simulink subsystem "SubFaultGate"  (R2026a)
settings: Solver=VariableStepAuto
settings Model: Creator=sarah  LastModifiedBy=sarah

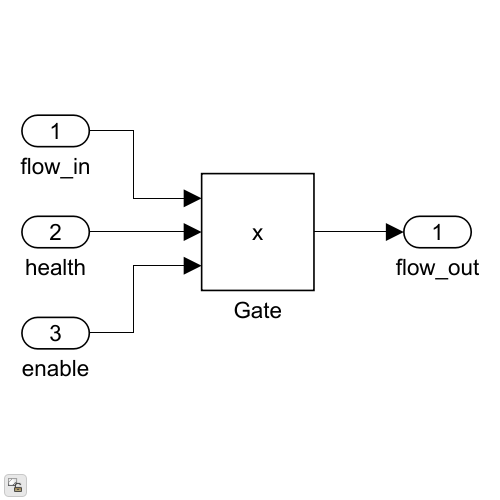
[thumbnail: Simulink's stored preview of the top-level diagram]
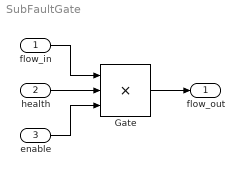
== system SubFaultGate ==
  flow_in : Inport
  health : Inport  Port=2
  enable : Inport  Port=3
  Gate : Product  Inputs=3
  flow_out : Outport
  wires:
  health/1 -> Gate/2
  flow_in/1 -> Gate/1
  Gate/1 -> flow_out/1
  enable/1 -> Gate/3
